simulink library "asbhl20scdexblks"  (R2016b)
settings: Solver=ode45  StartTime=0.0  StopTime=10.0  RelTol=1e-3
undefined symbols (not defined in the file): den, DiscIntNeverNeededParam, num
Description:
  | HL-20 lead-lag controller component module: discrete and continuous lead-lag controllers
settings Model: ExtModeAutoUpdateStatusClock=off  Creator=The MathWorks, Inc.  LastModifiedBy=The MathWorks, Inc.
settings DataIOCC: LimitDataPoints=on  SaveFormat=Array  SignalLoggingSaveFormat=ModelDataLogs
settings OptimizationCC: BlockReduction=off  BooleanDataType=off  ExpressionDepthLimit=2147483647  LifeSpan=inf
settings DebuggingCC: SaveWithParameterizedLinksMsg=none  UnderspecifiedInitializationDetection=Classic  MergeDetectMultiDrivingBlocksExec=none  SignalResolutionControl=TryResolveAllWithWarning  FcnCallInpInsideContextMsg=warning  AllowSymbolicDim=off  StateNameClashWarn=warning  StrictBusMsg=Warning  SFUnexpectedBacktrackingDiag=warning  SFNoUnconditionalDefaultTransitionDiag=warning  SFExecutionAtInitializationDiag=none
settings HardwareCC: ProdBitPerPointer=32  ProdBitPerSizeT=32  ProdBitPerPtrDiffT=32  ProdLargestAtomicFloat=None  ProdIntDivRoundTo=Undefined  ProdEndianess=Unspecified  ProdWordSize=32  ProdHWDeviceType=32-bit Generic  TargetUnknown=on
settings ModelReferenceCC: PropagateSignalLabelsOutOfModel=off
settings GRTTargetCC: TargetLangStandard=C89/C90 (ANSI)  GeneratePreprocessorConditionals=Disable all
settings ConfigComp: CovMetricSettings=dw  CovHtmlReporting=on  CovSaveCumulativeToWorkspaceVar=on  CovSaveSingleToWorkspaceVar=on  CovExternalEMLEnable=off

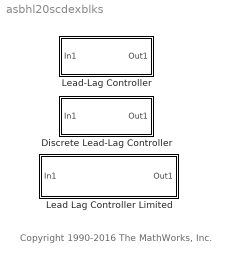
== system asbhl20scdexblks ==
  note: Copyright 1990-2016 The MathWorks, Inc.
  Discrete Lead-Lag Controller : Subsystem  SCDConfigFcn=scddleadexample  mask(Lead-Lag Controller){Zero=15, Pole=50, Ts=0.01}
      mask prompts: Zero "Zero Frequency (rad/s)"; Pole "Pole Frequency (rad/s)"; Ts "Sample Time"
      mask help: This block implements a lead-lag controller which consists of 1 zero, 1 pole, and a gain.
      mask init:
      | sys = c2d(tf([1/Zero 1],[1/Pole 1]),Ts);
      | [num,den] = tfdata(sys,'v');
      mask Display: dpoly([1/Zero 1],[1/Pole 1],'s')
  Lead Lag Controller Limited : Subsystem  mask{ZF=0.0400436516896399, PF=15.0000560854201, Ts=0, lower_limit=0, upper_limit=0}
      mask prompts: ZF "Zero Frequency (rad/s)"; PF "Pole  Frequency (rad/s)"; Ts "Sample Time"; lower_limit "Lower Limit"; upper_limit "Upper Limit"
      mask Display: text(0.01,0.5,'Lead-Lag Controller Limited')
  Lead-Lag Controller : Subsystem  SCDConfigFcn=scdleadexample  mask(Lead-Lag Controller){Gain=100, Zero=15, Pole=50}
      mask prompts: Zero "Zero Frequency (rad/s)"; Pole "Pole Frequency (rad/s)"
      mask help: This block implements a lead-lag controller which consists of 1 zero, 1 pole, and a gain.
      mask Display: fprintf('Lead-Lag Ctrl');

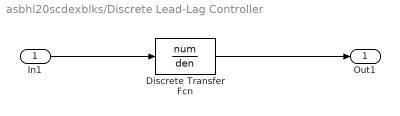
== system asbhl20scdexblks/Discrete Lead-Lag Controller ==
  In1 : Inport
  Discrete Transfer Fcn : DiscreteTransferFcn  Numerator=num  Denominator=den  SampleTime=Ts
  Out1 : Outport
  wires:
  Discrete Transfer Fcn/1 -> Out1/1
  In1/1 -> Discrete Transfer Fcn/1

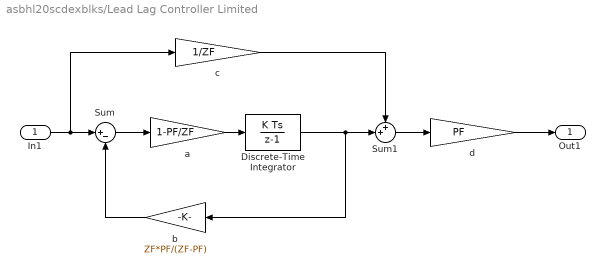
== system asbhl20scdexblks/Lead Lag Controller Limited ==
  In1 : Inport
  Discrete-Time Integrator : DiscreteIntegrator  SampleTime=Ts  LimitOutput=on  UpperSaturationLimit=upper_limit  LowerSaturationLimit=lower_limit  ICPrevOutput=DiscIntNeverNeededParam  ICPrevScaledInput=DiscIntNeverNeededParam
  Sum : Sum  Inputs=|+-
  Sum1 : Sum  Inputs=++|
  a : Gain  Gain=1-PF/ZF
  b : Gain  Gain=ZF*PF/(ZF-PF)
  c : Gain  Gain=1/ZF
  d : Gain  Gain=PF
  Out1 : Outport
  wires:
  In1/1 -> Sum/1, c/1
  Sum/1 -> a/1
  c/1 -> Sum1/1
  Sum1/1 -> d/1
  b/1 -> Sum/2
  d/1 -> Out1/1
  a/1 -> Discrete-Time Integrator/1
  Discrete-Time Integrator/1 -> Sum1/2, b/1

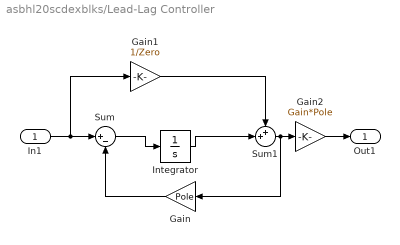
== system asbhl20scdexblks/Lead-Lag Controller ==
  In1 : Inport
  Gain : Gain  Gain=Pole
  Gain1 : Gain  Gain=1/Zero
  Gain2 : Gain  Gain=Gain*Pole
  Integrator : Integrator
  Sum : Sum  Inputs=|+-
  Sum1 : Sum  Inputs=++|
  Out1 : Outport
  wires:
  Sum1/1 -> Gain/1, Gain2/1
  Integrator/1 -> Sum1/2
  Gain1/1 -> Sum1/1
  Sum/1 -> Integrator/1
  In1/1 -> Sum/1, Gain1/1
  Gain/1 -> Sum/2
  Gain2/1 -> Out1/1
